simulink model "toUdp"  (R2017b)
settings: Solver=ode3  StartTime=0.0  StopTime=inf  FixedStep=0.01  RelTol=1e-3  EnableMultiTasking=on
model workspace (MAT data in the model file):
  SL_ROS_VariableLengthArrays_MaxSizes.CommonInfo.ArrayTruncateAction = 'EmitWarning'
  SL_ROS_VariableLengthArrays_MaxSizes.MsgTypeMap = containers.Map
  SL_ROS_VariableLengthArrays_MaxSizes.MsgTypeMap.serialization.keys = {'std_msgs/Float32MultiArray'}
  SL_ROS_VariableLengthArrays_MaxSizes.MsgTypeMap.serialization.values{1}.PropertyName = 'Data'
  SL_ROS_VariableLengthArrays_MaxSizes.MsgTypeMap.serialization.values{1}.DataType = 'single'
  SL_ROS_VariableLengthArrays_MaxSizes.MsgTypeMap.serialization.values{1}.MaxLength = 2
  SL_ROS_VariableLengthArrays_MaxSizes.MsgTypeMap.serialization.uniformity = 0
  SL_ROS_VariableLengthArrays_MaxSizes.MsgTypeMap.serialization.keyType = 'char'
  SL_ROS_VariableLengthArrays_MaxSizes.MsgTypeMap.serialization.valueType = 'any'
libraries: robotlib x3, etargetslib x2, dspnetwork x2
settings Model: Creator=Centauro  LastModifiedBy=antonio
settings DataIOCC: LimitDataPoints=on  SaveFormat=Array
settings OptimizationCC: PassReuseOutputArgsThreshold=0  MaxStackSize=64
settings DebuggingCC: ParameterTunabilityLossMsg=error  SFUnexpectedBacktrackingDiag=warning  SFNoUnconditionalDefaultTransitionDiag=warning  SFExecutionAtInitializationDiag=none
settings HardwareCC: ProdBitPerPointer=32  ProdBitPerSizeT=32  ProdBitPerPtrDiffT=32  ProdLargestAtomicFloat=None  ProdIntDivRoundTo=Undefined  ProdEndianess=Unspecified  ProdWordSize=32  ProdHWDeviceType=Generic->Unspecified (assume 32-bit Generic)  UseEmbeddedCoderFeatures=off
settings ModelReferenceCC: PropagateSignalLabelsOutOfModel=off
settings SFSimCC: MATLABDynamicMemAlloc=off
settings RTWCC: SystemTargetFile=ert.tlc  HardwareBoard=Robot Operating System (ROS)  TemplateMakefile=ert_default_tmf  GenerateReport=on  Toolchain=Catkin  LaunchReport=on  TargetLang=C++
settings CodeAppCC: ForceParamTrailComments=on  OperatorAnnotations=on
settings ERTTargetCC: ERTCustomFileBanners=off  SupportContinuousTime=on  SupportNonInlinedSFcns=on  RemoveResetFunc=off  ModelStepFunctionPrototypeControlCompliant=off
settings ConfigComp: CovMetricSettings=dw  CovHtmlReporting=on  CovSaveCumulativeToWorkspaceVar=on  CovSaveSingleToWorkspaceVar=on  CovExternalEMLEnable=off

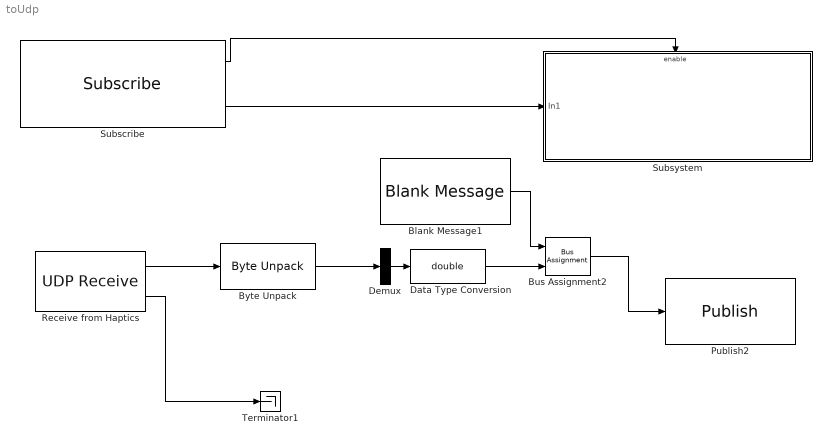
== system toUdp ==
  Blank Message1 : robotlib/Blank Message  SourceLibraryInfo=This block requires Robotics System Toolbox  messageType=std_msgs/Float64  SampleTime=inf
      settings: SourceProductBaseCode=RO
  Bus Assignment2 : BusAssignment  AssignedSignals=Data
  Byte Unpack : etargetslib/Byte Unpack  dimensions={[1]}  datatypes={'single'}  byteAlign=1
  Data Type Conversion : DataTypeConversion  OutDataTypeStr=double
  Demux : Demux  Outputs=[1]
  Publish2 : robotlib/Publish  SourceLibraryInfo=This block requires Robotics System Toolbox  topicSource=Select from ROS network  topic=/left_hand/force_ref  messageType=std_msgs/Float64  messageQueueLength=1
      settings: SourceProductBaseCode=RO
  Receive from Haptics : dspnetwork/UDP Receive  localURL='0.0.0.0'  localPort=17006  remoteURL='10.24.4.10'  remotePort=-1  recvBufferSize=1*4  dims=1*4  signalDatatype=uint8  isVarSize=off  showBlockingTime=on  blockingTime=0.01  sampletime=0.01  blockPlatform=HOST
      settings: SourceProductName=DSP System Toolbox  SourceProductBaseCode=DS
  Subscribe : robotlib/Subscribe  SourceLibraryInfo=This block requires Robotics System Toolbox  topicSource=Select from ROS network  topic=/left_hand/position_curr  messageType=std_msgs/Float64  sampleTime=0.01  messageQueueLength=1
      settings: SourceProductBaseCode=RO
  Subsystem : Subsystem
  Terminator1 : Terminator
  wires:
  Subscribe/1 -> Subsystem/Enable
  Byte Unpack/1 -> Demux/1
  Receive from Haptics/1 -> Byte Unpack/1
  Receive from Haptics/2 -> Terminator1/1
  Subscribe/2 -> Subsystem/1(In1)
  Demux/1 -> Data Type Conversion/1
  Bus Assignment2/1 -> Publish2/1
  Blank Message1/1 -> Bus Assignment2/1
  Data Type Conversion/1 -> Bus Assignment2/2

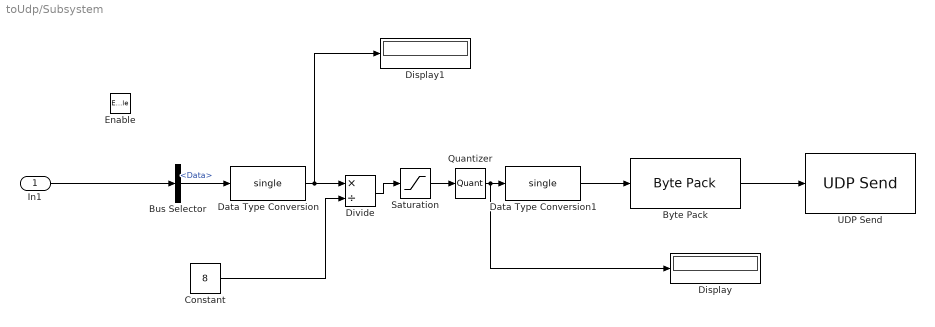
== system toUdp/Subsystem ==
  In1 : Inport
  Enable : EnablePort
  Bus Selector : BusSelector  OutputSignals=Data
  Byte Pack : etargetslib/Byte Pack  datatypes={'single'}  byteAlign=1
  Constant : Constant  Value=8  OutDataTypeStr=single
  Data Type Conversion : DataTypeConversion  OutDataTypeStr=single
  Data Type Conversion1 : DataTypeConversion  OutDataTypeStr=single
  Display : Display
  Display1 : Display
  Divide : Product  Inputs=*/
  Quantizer : Quantizer  QuantizationInterval=0.1
  Saturation : Saturate  UpperLimit=1  LowerLimit=0
  UDP Send : dspnetwork/UDP Send  remoteURL='10.24.4.10'  remotePort=17106  localURL='0.0.0.0'  localPortSource=Automatically determine  localPort=-1  sampletime=-1  blockPlatform=HOST  separateLengthPort=0
      settings: SourceProductName=DSP System Toolbox  SourceProductBaseCode=DS
  wires:
  In1/1 -> Bus Selector/1
  Bus Selector/1 -> Data Type Conversion/1  "<Data>"
  Byte Pack/1 -> UDP Send/1
  Data Type Conversion/1 -> Display1/1, Divide/1
  Divide/1 -> Saturation/1
  Constant/1 -> Divide/2
  Data Type Conversion1/1 -> Byte Pack/1
  Saturation/1 -> Quantizer/1
  Quantizer/1 -> Display/1, Data Type Conversion1/1
